simulink model "ILRF"  (R2023a)
settings: Solver=VariableStepAuto  StartTime=0.0  StopTime=10.0  RelTol=1e-3
values from neighbouring files (symbols this model uses):
  b = 0.490    (= 0.49)    [Cascaded_PI_Step.m]    (also in Cascaded_PI_Zero_Ref.m; Gain_Scheduled_PI_Step.m; Gain_Scheduled_PI_Zero_Ref.m; Inner_Loop_Relay_Feedback.m)
  Clda = 0.65    [Cascaded_PI_Step.m]    (also in Cascaded_PI_Zero_Ref.m; Gain_Scheduled_PI_Step.m; Gain_Scheduled_PI_Zero_Ref.m; Inner_Loop_Relay_Feedback.m)
  Clo = 1.108    [Cascaded_PI_Step.m]    (also in Cascaded_PI_Zero_Ref.m; Gain_Scheduled_PI_Step.m; Gain_Scheduled_PI_Zero_Ref.m; Inner_Loop_Relay_Feedback.m)
  Clp = -1.5    [Cascaded_PI_Step.m]    (also in Cascaded_PI_Zero_Ref.m = -11.5; Gain_Scheduled_PI_Step.m = -11.5; Gain_Scheduled_PI_Zero_Ref.m = -11.5; Inner_Loop_Relay_Feedback.m = -11.5)
  Kp = 0.3    [Inner_Loop_Relay_Feedback.m]
  p_des = 100    [Inner_Loop_Relay_Feedback.m]
  rho = 1.204    [Cascaded_PI_Step.m]    (also in Cascaded_PI_Zero_Ref.m; Gain_Scheduled_PI_Step.m; Gain_Scheduled_PI_Zero_Ref.m; Inner_Loop_Relay_Feedback.m)
  S = 0.44    [Cascaded_PI_Step.m]    (also in Cascaded_PI_Zero_Ref.m; Gain_Scheduled_PI_Step.m; Gain_Scheduled_PI_Zero_Ref.m; Inner_Loop_Relay_Feedback.m)
  Va = 15    [Cascaded_PI_Step.m]    (also in Cascaded_PI_Zero_Ref.m; Gain_Scheduled_PI_Step.m; Gain_Scheduled_PI_Zero_Ref.m; Inner_Loop_Relay_Feedback.m)
settings Model: Creator=brend  LastModifiedBy=brend

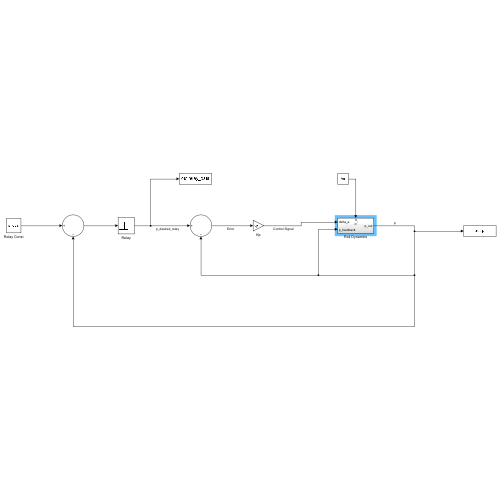
[thumbnail: Simulink's stored preview of the top-level diagram]
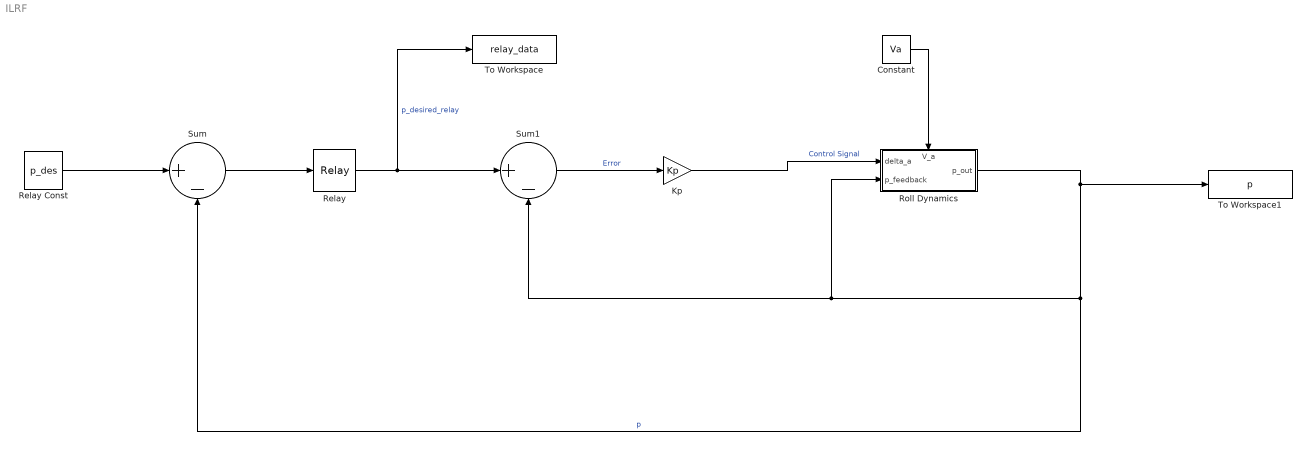
== system ILRF ==
  Constant : Constant  Value=Va
  Kp : Gain  Gain=Kp
  Relay : Relay  OnSwitchValue=130  OffSwitchValue=70  OnOutputValue=p_des  OffOutputValue=-p_des
  Relay Const : Constant  Value=p_des
  Roll Dynamics : Subsystem
      settings: PortSchema="{\"entries\":[{\"content\":{\"sides\":[{\"content\":{\"connectorIds\":[\"In1\",\"In2\"]},\"type\":\"ConnectorPlacement.EquallySpacedRectSide\",\"uuid\":\"0ac85a74-38c1-4d65-b1c0-9ca36de2cddb\"},{\"content\":{\"connectorIds\":[\"Out1\"],\"side\":\"RIGHT\"},\"type\":\"ConnectorPlacement.EquallySpacedRectSide\",\"uuid\":\"84e324c4-b4ec-429b-b00b-3022433bb281\"},{\"content\":{\"connectorIds\":[\"In3\"],\"side\":\"TOP\"},\"type\":\"ConnectorPlacement.EquallySpacedRectSide\",\"uuid\":\"b4486eb0-6e0f-4f77-80f0-5dbcf5ffe993\"}]},\"type\":\"ConnectorPlacement.EquallySpacedConnector\",\"uuid\":\"7fd31f13-990e-44ec-9889-e700ea070706\"}],\"packageUris\":[\"http://schema.mathworks.com/mf0/Connector/R2020b\"],\"version\":\"1.0\"}"
  Sum : Sum  Inputs=|+-
  Sum1 : Sum  Inputs=|+-
  To Workspace : ToWorkspace  VariableName=relay_data  SaveFormat=Timeseries  SampleTime=-1
  To Workspace1 : ToWorkspace  VariableName=p  SaveFormat=Timeseries  SampleTime=-1
  wires:
  Relay Const/1 -> Sum/1
  Sum/1 -> Relay/1
  Relay/1 -> To Workspace/1, Sum1/1  "p_desired_relay"
  Sum1/1 -> Kp/1  "Error"
  Kp/1 -> Roll Dynamics/1(delta_a)  "Control Signal"
  Roll Dynamics/1(p_out) -> To Workspace1/1, Roll Dynamics/2(p_feedback), Sum1/2, Sum/2  "p"
  Constant/1 -> Roll Dynamics/3(V_a)

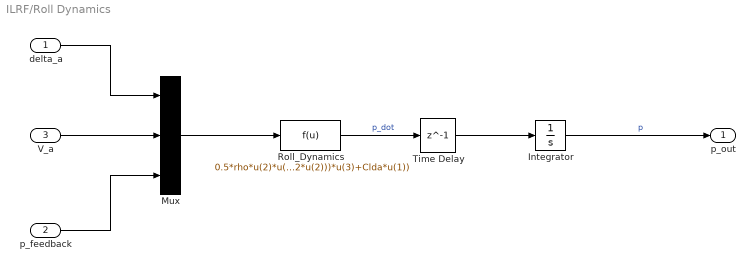
== system ILRF/Roll Dynamics ==
  delta_a : Inport
  p_feedback : Inport  Port=2
  V_a : Inport  Port=3
  Integrator : Integrator
  Mux : Mux  Inputs=3
  Roll_Dynamics : Fcn  Expr=0.5*rho*u(2)*u(2)*S*b*(Clo + Clp*(b/(2*u(2)))*u(3)+Clda*u(1))
  Time Delay : Delay  DelayLength=1
  p_out : Outport
  wires:
  delta_a/1 -> Mux/1
  Mux/1 -> Roll_Dynamics/1
  Integrator/1 -> p_out/1  "p"
  V_a/1 -> Mux/2
  p_feedback/1 -> Mux/3
  Roll_Dynamics/1 -> Time Delay/1  "p_dot"
  Time Delay/1 -> Integrator/1
